simulink model "NL_PID_B0_fhan_MODEL"  (Simulink 7.6)
settings: Solver=ode45  StartTime=0.0  StopTime=20  RelTol=1e-3
settings Model: Creator=Administrator  LastModifiedBy=Administrator
settings DebuggingCC: SolverPrmCheckMsg=none

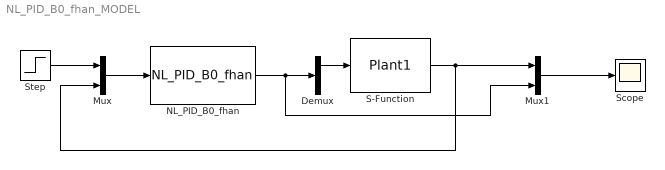
== system NL_PID_B0_fhan_MODEL ==
  Demux : Demux  Outputs=2
  Mux : Mux  Inputs=2
  Mux1 : Mux  Inputs=2
  NL_PID_B0_fhan : S-Function  FunctionName=NL_PID_B0_fhan  Parameters=r0,h0,r1,h1,h,Bet0,r2,h2  EnableBusSupport=off  mask{r0=0.5, h0=0.01, r1=30, h1=0.01, h=0.01, Bet0=500, r2=20, h2=0.08}
      mask prompts: r0 "r0="; r1 "r1="; h1 "h1="; h "h="; Bet0 "Bet0="; r2 "r2="; h2 "h2="
  S-Function : S-Function  FunctionName=Plant1  EnableBusSupport=off
  Scope : Scope
      settings: YMin=-2.75  YMax=1.25
  Step : Step  Time=0  SampleTime=0
  wires:
  Step/1 -> Mux/1
  Mux/1 -> NL_PID_B0_fhan/1
  Mux1/1 -> Scope/1
  NL_PID_B0_fhan/1 -> Demux/1, Mux1/2
  Demux/1 -> S-Function/1
  S-Function/1 -> Mux1/1, Mux/2
